simulink model "controller_velocity"  (R2021a)
settings: Solver=FixedStepAuto  StartTime=0.0  StopTime=10.0  FixedStep=1/sim_freq  RelTol=1e-3
undefined symbols (not defined in the file): Ts_pos_control
settings Model: Creator=francois  LastModifiedBy=esl
settings SolverCC: ZeroCrossControl=DisableAll  AlgebraicLoopSolver=TrustRegion
settings DataIOCC: SaveOutput=off  SaveTime=off
settings DebuggingCC: ModelReferenceExtraNoncontSigs=none  SFMachineParentedDataDiag=warning
settings ModelReferenceCC: ModelReferenceNumInstancesAllowed=Single
settings GRTTargetCC: CombineOutputUpdateFcns=off  MatFileLogging=off

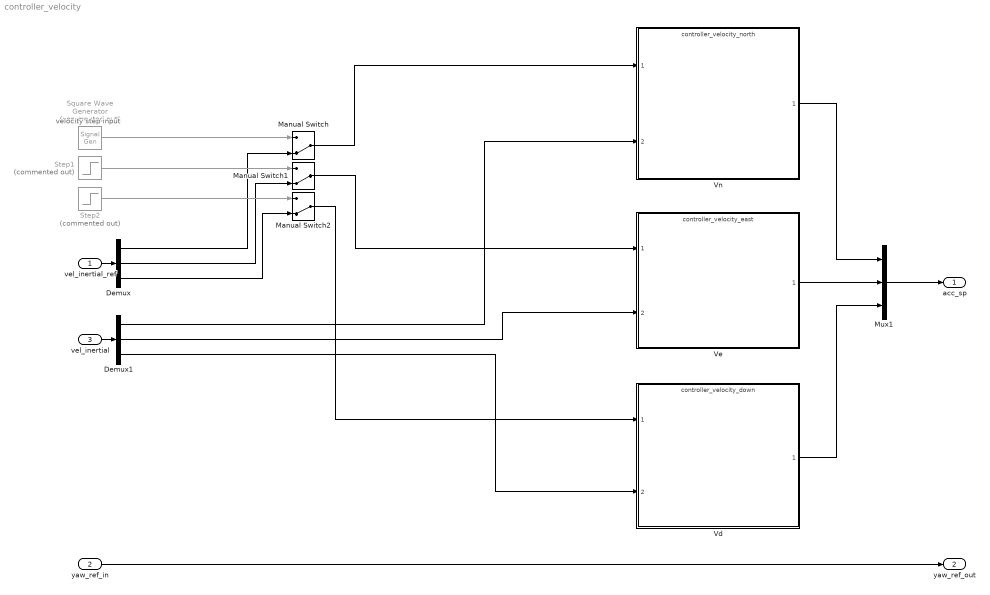
== system controller_velocity ==
  note: velocity step input
  "vel_inertial_ref " : Inport  SampleTime=Ts_pos_control
  yaw_ref_in : Inport  Port=2  SampleTime=Ts_pos_control
  "vel_inertial " : Inport  Port=3  SampleTime=Ts_pos_control
  Demux : Demux  Outputs=3
  Demux1 : Demux  Outputs=3
  Manual Switch : ManualSwitch  CurrentSetting=0
  Manual Switch1 : ManualSwitch  CurrentSetting=0
  Manual Switch2 : ManualSwitch  CurrentSetting=0
  Mux1 : Mux  Inputs=3
  Square Wave Generator : SignalGenerator  Commented=on  WaveForm=square  Amplitude=0.5  Frequency=0.1  Units=rad/sec
  Step1 : Step  Commented=on  Time=80  SampleTime=0
  Step2 : Step  Commented=on  After=0  SampleTime=0
  Vd : ModelReference  ModelNameDialog=controller_velocity_down.slx  SimulationMode=Normal  ModelReferenceVersion=3.4
  Ve : ModelReference  ModelNameDialog=controller_velocity_east.slx  SimulationMode=Normal  ModelReferenceVersion=3.3
  Vn : ModelReference  ModelNameDialog=controller_velocity_north.slx  SimulationMode=Normal  ModelReferenceVersion=3.3
  acc_sp : Outport
  "yaw_ref_out " : Outport  Port=2
  wires:
  "vel_inertial "/1 -> Demux1/1
  yaw_ref_in/1 -> "yaw_ref_out "/1
  Demux1/2 -> Ve/2
  Demux1/1 -> Vn/2
  Demux1/3 -> Vd/2
  "vel_inertial_ref "/1 -> Demux/1
  Demux/3 -> Manual Switch2/2
  Demux/2 -> Manual Switch1/2
  Demux/1 -> Manual Switch/2
  Square Wave Generator/1 -> Manual Switch/1
  Step1/1 -> Manual Switch1/1
  Step2/1 -> Manual Switch2/1
  Manual Switch/1 -> Vn/1
  Manual Switch1/1 -> Ve/1
  Manual Switch2/1 -> Vd/1
  Vn/1 -> Mux1/1
  Ve/1 -> Mux1/2
  Vd/1 -> Mux1/3
  Mux1/1 -> acc_sp/1
